simulink model "TPI_PLL"  (R2015b)
settings: Solver=FixedStepAuto  SolverMode=SingleTasking  StartTime=0.0  StopTime=3  FixedStep=Ts  RelTol=1e-3
values from neighbouring files (symbols this model uses):
  fpScan = 0    [TPI_PLL_m.m]
  idref = 10    [TPI_PLL_m.m]
  iqref = 0    [TPI_PLL_m.m]
  Ki_PLL = (-2*xi^2*omegaPLL^2+omegaPLL^2*sqrt(1+4*xi^4))/V1    [TPI_PLL_m.m]
  Kii = 1    [TPI_PLL_m.m]
  Kp_PLL = sqrt(4*xi^2*Ki_PLL/V1)    [TPI_PLL_m.m]
  Kpi = 0.1    [TPI_PLL_m.m]
  PhaseB = 0    [TPI_PLL_m.m]
  PhaseC = 0    [TPI_PLL_m.m]
  Ts = 1e-4    (= 0.0001)    [TPI_PLL_m.m]
  Udc = 400    [TPI_PLL_m.m]
  UpScan = 0    [TPI_PLL_m.m]
libraries: powerlib x15, powerlib_meascontrol x7, simulink x1
Description:
  | Copyright 2008-2015 The MathWorks, Inc.
settings Model: ExtModeTrigMode=oneshot  ExtModeArmWhenConnect=off  ExtModeAutoUpdateStatusClock=off  Creator=MathWorks  LastModifiedBy=Tommy
settings DataIOCC: LimitDataPoints=off  SaveFormat=StructureWithTime  SignalLoggingSaveFormat=ModelDataLogs  SignalLogging=off  DSMLogging=off  SaveTime=off  SignalLoggingName=sigsOut
settings OptimizationCC: BlockReduction=off  BooleanDataType=off  ExpressionDepthLimit=2147483647  InitFltsAndDblsToZero=on  EfficientMapNaN2IntZero=off
settings DebuggingCC: SaveWithParameterizedLinksMsg=none  UnderspecifiedInitializationDetection=Classic  MergeDetectMultiDrivingBlocksExec=none  CheckExecutionContextPreStartOutputMsg=on  CheckExecutionContextRuntimeOutputMsg=on  SignalResolutionControl=TryResolveAllWithWarning  MultiTaskDSMMsg=warning  MultiTaskCondExecSysMsg=none  FcnCallInpInsideContextMsg=UseLocalSettings  StateNameClashWarn=warning
settings HardwareCC: ProdBitPerPointer=32  ProdLargestAtomicFloat=None  ProdIntDivRoundTo=Undefined  ProdEndianess=Unspecified  ProdWordSize=32  ProdHWDeviceType=32-bit Generic  TargetUnknown=on
settings GRTTargetCC: TargetFcnLib=ansi_tfl_tmw.mat  GeneratePreprocessorConditionals=Disable all  CombineOutputUpdateFcns=off  GRTInterface=on
settings ConfigComp: CovModelRefEnable=Off  CovSFcnEnable=off

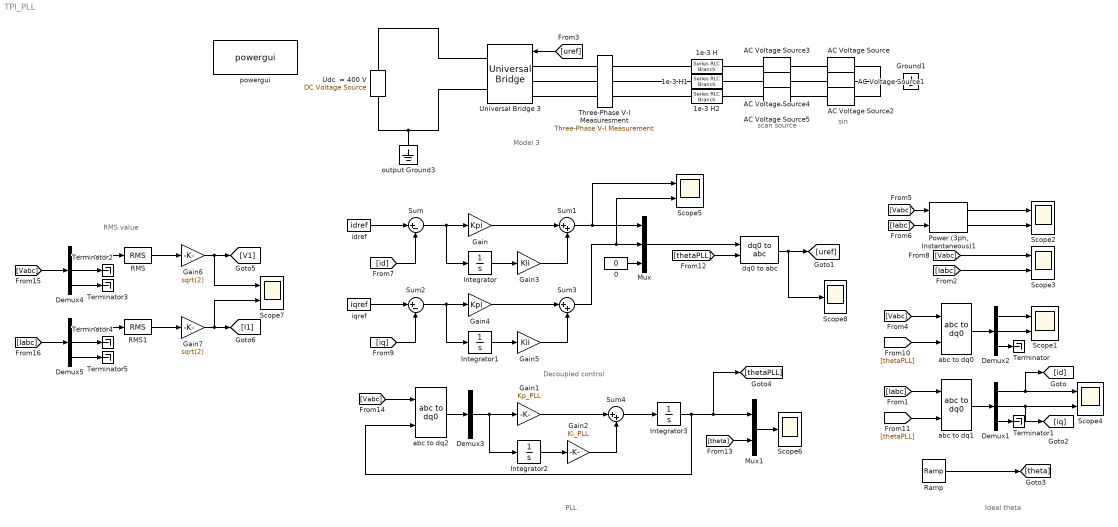
== system TPI_PLL ==
  note: scan source
  note: RMS value
  note: Decoupled control
  note: sin
  note: Model 3
  note: PLL
  note: Ideal theta
  0 : Constant  Value=0
  1e-3 H : powerlib/Elements/Series RLC Branch  LConnTagsString=__new0  RConnTagsString=__new0  BranchType=R  Resistance=1e-3  Inductance=1e-3  SetiL0=off  InitialCurrent=0  Capacitance=1e-6  Setx0=off  InitialVoltage=0  Measurements=None
  1e-3 H1 : powerlib/Elements/Series RLC Branch  LConnTagsString=__new0  RConnTagsString=__new0  BranchType=R  Resistance=1e-3  Inductance=1e-3  SetiL0=off  InitialCurrent=0  Capacitance=1e-6  Setx0=off  InitialVoltage=0  Measurements=None
  1e-3 H2 : powerlib/Elements/Series RLC Branch  LConnTagsString=__new0  RConnTagsString=__new0  BranchType=R  Resistance=1e-3  Inductance=1e-3  SetiL0=off  InitialCurrent=0  Capacitance=1e-6  Setx0=off  InitialVoltage=0  Measurements=None
  AC Voltage Source : powerlib/Electrical Sources/AC Voltage Source  Amplitude=100  Phase=0  Frequency=50  SampleTime=Ts  Measurements=None  BusType=swing  Pref=10e3  Qref=0  Qmin=-inf  Qmax=+inf
  AC Voltage Source1 : powerlib/Electrical Sources/AC Voltage Source  Amplitude=100  Phase=-120  Frequency=50  SampleTime=Ts  Measurements=None  BusType=swing  Pref=10e3  Qref=0  Qmin=-inf  Qmax=+inf
  AC Voltage Source2 : powerlib/Electrical Sources/AC Voltage Source  Amplitude=100  Phase=120  Frequency=50  SampleTime=Ts  Measurements=None  BusType=swing  Pref=10e3  Qref=0  Qmin=-inf  Qmax=+inf
  AC Voltage Source3 : powerlib/Electrical Sources/AC Voltage Source  Amplitude=UpScan  Phase=0  Frequency=fpScan  SampleTime=Ts  Measurements=None  BusType=swing  Pref=10e3  Qref=0  Qmin=-inf  Qmax=+inf
  AC Voltage Source4 : powerlib/Electrical Sources/AC Voltage Source  Amplitude=UpScan  Phase=PhaseB  Frequency=fpScan  SampleTime=Ts  Measurements=None  BusType=swing  Pref=10e3  Qref=0  Qmin=-inf  Qmax=+inf
  AC Voltage Source5 : powerlib/Electrical Sources/AC Voltage Source  Amplitude=UpScan  Phase=PhaseC  Frequency=fpScan  SampleTime=Ts  Measurements=None  BusType=swing  Pref=10e3  Qref=0  Qmin=-inf  Qmax=+inf
  Demux{1..5} (5 alike) : Demux  Outputs=3
  Gain : Gain  Gain=Kpi
  Gain1 : Gain  Gain=Kp_PLL
  Gain2 : Gain  Gain=Ki_PLL
  Gain3 : Gain  Gain=Kii
  Gain4 : Gain  Gain=Kpi
  Gain5 : Gain  Gain=Kii
  Gain6 : Gain  Gain=sqrt(2)
  Gain7 : Gain  Gain=sqrt(2)
  Ground1 : powerlib/Elements/Ground  LConnTagsString=a
  Integrator{,1..3} (4 alike) : Integrator  UpperSaturationLimit=50  LowerSaturationLimit=-50
  Mux : Mux  Inputs=3
  Mux1 : Mux  Inputs=2
  "Power (3ph, Instantaneous)1" : powerlib_meascontrol/Measurements/Power (3ph, Instantaneous)
  RMS : powerlib_meascontrol/Measurements/RMS  TrueRMS=on  Freq=50  RMSInit=0  Ts=0
  RMS1 : powerlib_meascontrol/Measurements/RMS  TrueRMS=on  Freq=50  RMSInit=0  Ts=0
  Ramp : simulink/Sources/Ramp  slope=2*pi*50  start=0  X0=0
  Scope{1..5,7} (6 alike) : Scope  NumInputPorts=2
  Scope6 : Scope
  Scope8 : Scope
  Sum : Sum  Inputs=|+-
  Sum1 : Sum  Inputs=|++
  Sum2 : Sum  Inputs=|+-
  Sum3 : Sum  Inputs=|++
  Sum4 : Sum  Inputs=|++
  Terminator{,1..5} (6 alike) : Terminator
  Three-Phase V-I Measuresment : powerlib/Measurements/Three-Phase V-I Measurement  VoltageMeasurement=phase-to-ground  SetLabelV=on  LabelV=Vabc  Vpu=off  VpuLL=off  CurrentMeasurement=yes  SetLabelI=on  LabelI=Iabc  Ipu=off  Pbase=100e6  Vbase=500e3  OutputType=Complex  PhasorSimulation=off  PSBequivalent=0
  Udc  = 400 V : powerlib/Electrical Sources/DC Voltage Source  Description=source block  Amplitude=Udc  Measurements=None
      settings: AttributesFormatString=\n
  Universal Bridge 3 : powerlib/Power Electronics/Universal Bridge  Arms=3  SnubberResistance=10000  SnubberCapacitance=inf  Device=Average-model based VSC  Ron=1e-4  Lon=0  ForwardVoltages="[  1  1  ]"  ForwardVoltage=.8  GTOparameters=[ 10e-6 , 20e-6 ]  IGBTparameters=[ 1e-6 , 2e-6 ]  Measurements=None  Measurements_2=None  converterType=Rectifier
      settings: AttributesFormatString=Device: %<Device>
  abc to dq0 : powerlib_meascontrol/Transformations/abc to dq0  Alignment=90 degrees behind phase A axis
  abc to dq1 : powerlib_meascontrol/Transformations/abc to dq0  Alignment=90 degrees behind phase A axis
  abc to dq2 : powerlib_meascontrol/Transformations/abc to dq0  Alignment=90 degrees behind phase A axis
  dq0 to abc : powerlib_meascontrol/Transformations/dq0 to abc  Alignment=90 degrees behind phase A axis
  idref : Constant  Value=idref
  "iqref " : Constant  Value=iqref
  output Ground3 : powerlib/Elements/Ground  LConnTagsString=a
  powergui : powerlib/powergui  Priority=2  SimulationMode=Discrete  SolverType=Tustin  SampleTime=100e-6  frequency=60  SPID=off  DisableSnubberDevices=off  DisableRonSwitches=off  DisableVfSwitches=off  SwTol=0  DisplayEquations=off  Interpol=off  ExternalGateDelay=off  methode=off  Ts=0  FunctionMessages=off  echomessages=off  HookPort=off  EnableUseOfTLC=off  x0status=blocks  frequencyindice=50  Pbase=100e6  ErrMax=1e-4  Iterations=50  UnitsV=kV  UnitsW=MW  buscounter=0  RestoreLinks=warning  ResistiveCurrentMeasurement=off  Frange=[0:2:500]  Ylog=off  Xlog=off  ShowGrid=off  save=off  variable=ZData  structure=UI  ZoomFFT=off  StartTime=2  cycles=50  DisplayStyle=2  fundamental=50  FreqAxis=off  MaxFrequency=5000  frequencyindicesteady=1  RmsSteady=1  display=off
  wires:
  [Vabc] -> abc to dq0/1
  abc to dq0/1 -> Demux2/1
  Demux2/2 -> Scope1/2
  Demux2/1 -> Scope1/1
  [uref] -> Universal Bridge 3/1
  [Iabc] -> abc to dq1/1
  abc to dq1/1 -> Demux1/1
  Demux1/2 -> [iq], Scope4/2
  Demux1/1 -> [id], Scope4/1
  [id] -> Sum/2
  idref/1 -> Sum/1
  Sum/1 -> Gain/1, Integrator/1
  Integrator/1 -> Gain3/1
  Gain/1 -> Sum1/1
  Gain3/1 -> Sum1/2
  [iq] -> Sum2/2
  "iqref "/1 -> Sum2/1
  Sum2/1 -> Gain4/1, Integrator1/1
  Integrator1/1 -> Gain5/1
  Gain4/1 -> Sum3/1
  Gain5/1 -> Sum3/2
  Sum1/1 -> Scope5/1, Mux/1
  Sum3/1 -> Scope5/2, Mux/2
  0/1 -> Mux/3
  Mux/1 -> dq0 to abc/1
  Ramp/1 -> [theta]
  [thetaPLL] -> abc to dq0/2
  [thetaPLL] -> abc to dq1/2
  [thetaPLL] -> dq0 to abc/2
  dq0 to abc/1 -> Scope8/1, [uref]
  [Vabc] -> abc to dq2/1
  Integrator2/1 -> Gain2/1
  Gain1/1 -> Sum4/1
  Gain2/1 -> Sum4/2
  Sum4/1 -> Integrator3/1
  Integrator3/1 -> abc to dq2/2, [thetaPLL], Mux1/1
  abc to dq2/1 -> Demux3/1
  Demux3/2 -> Integrator2/1, Gain1/1
  Mux1/1 -> Scope6/1
  [theta] -> Mux1/2
  Demux2/3 -> Terminator/1
  Demux1/3 -> Terminator1/1
  [Vabc] -> Demux4/1
  Demux4/2 -> Terminator2/1
  Demux4/3 -> Terminator3/1
  Demux4/1 -> RMS/1
  RMS/1 -> Gain6/1
  Gain6/1 -> Scope7/1, [V1]
  [Iabc] -> Demux5/1
  Demux5/2 -> Terminator4/1
  Demux5/3 -> Terminator5/1
  Demux5/1 -> RMS1/1
  RMS1/1 -> Gain7/1
  Gain7/1 -> Scope7/2, [I1]
  [Vabc] -> Scope3/1
  [Iabc] -> "Power (3ph, Instantaneous)1"/2
  "Power (3ph, Instantaneous)1"/2 -> Scope2/2
  [Vabc] -> "Power (3ph, Instantaneous)1"/1
  "Power (3ph, Instantaneous)1"/1 -> Scope2/1
  [Iabc] -> Scope3/2
  connections:
  AC Voltage Source/LConn1 -- AC Voltage Source2/LConn1 -- Ground1/LConn1 -- AC Voltage Source1/LConn1
  Udc  = 400 V/LConn1 -- Universal Bridge 3/RConn2 -- output Ground3/LConn1
  Udc  = 400 V/RConn1 -- Universal Bridge 3/RConn1
  Three-Phase V-I Measuresment/LConn1 -- Universal Bridge 3/LConn1
  Three-Phase V-I Measuresment/LConn2 -- Universal Bridge 3/LConn2
  Three-Phase V-I Measuresment/LConn3 -- Universal Bridge 3/LConn3
  Three-Phase V-I Measuresment/RConn1 -- 1e-3 H/LConn1
  Three-Phase V-I Measuresment/RConn2 -- 1e-3 H1/LConn1
  Three-Phase V-I Measuresment/RConn3 -- 1e-3 H2/LConn1
  AC Voltage Source3/LConn1 -- AC Voltage Source/RConn1
  AC Voltage Source4/LConn1 -- AC Voltage Source1/RConn1
  AC Voltage Source5/LConn1 -- AC Voltage Source2/RConn1
  AC Voltage Source5/RConn1 -- 1e-3 H2/RConn1
  AC Voltage Source4/RConn1 -- 1e-3 H1/RConn1
  AC Voltage Source3/RConn1 -- 1e-3 H/RConn1
